simulink model "Top_Level_Model_arch"  (R2023a)
settings: Solver=VariableStepAuto  StartTime=0.0  StopTime=10.0  RelTol=1e-3
settings Model: Creator=hunte  LastModifiedBy=hunte

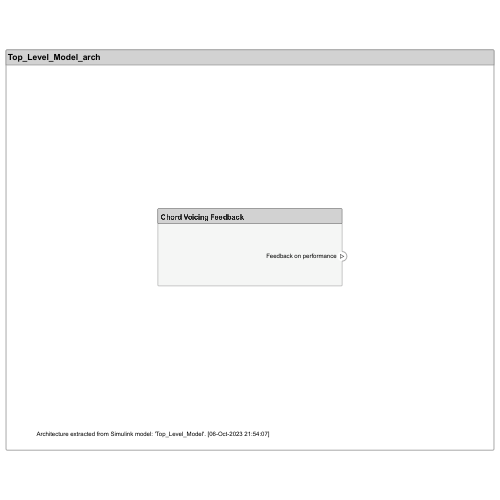
[thumbnail: Simulink's stored preview of the top-level diagram]
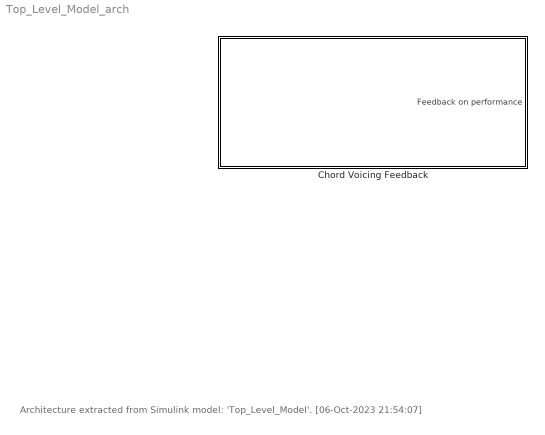
== system Top_Level_Model_arch ==
  note: Architecture extracted from Simulink model: 'Top_Level_Model'. [06-Oct-2023 21:54:07]
  "Chord Voicing Feedback " : Subsystem
      settings: PortSchema="{\"entries\":[{\"content\":{\"headerSize\":26,\"margin\":15,\"minimumSpacing\":25,\"sides\":[{\"content\":{},\"type\":\"ConnectorPlacement.EquallySpacedRectSide\",\"uuid\":\"aa7799b5-9463-4594-9ae2-36d4855ee31b\"},{\"content\":{\"connectorIds\":[\"Out1\"],\"side\":\"RIGHT\"},\"type\":\"ConnectorPlacement.EquallySpacedRectSide\",\"uuid\":\"2092a70f-f0fd-429a-8afe-090859a2b818\"},{\"content\":{\"side\":\"TOP\"},\"type\":\"ConnectorPlacement.EquallySpacedRectSide\",\"uuid\":\"da8f9889-6f26-4414-a897-b29829a1673f\"}]},\"type\":\"ConnectorPlacement.EquallySpacedConnector\",\"uuid\":\"7a26612b-cf01-40dc-98f5-e18304675eaa\"}],\"packageUris\":[\"http://schema.mathworks.com/mf0/Connector/R2020b\"],\"version\":\"1.0\"}"

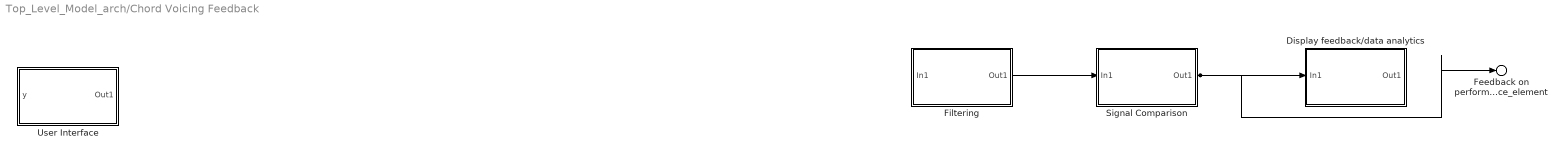
== system Top_Level_Model_arch/Chord Voicing Feedback  ==
  Display feedback/data analytics : Subsystem
      settings: PortSchema="{\"entries\":[{\"content\":{\"headerSize\":26,\"margin\":15,\"minimumSpacing\":25,\"sides\":[{\"content\":{\"connectorIds\":[\"In1\"]},\"type\":\"ConnectorPlacement.EquallySpacedRectSide\",\"uuid\":\"aa7799b5-9463-4594-9ae2-36d4855ee31b\"},{\"content\":{\"connectorIds\":[\"Out1\"],\"side\":\"RIGHT\"},\"type\":\"ConnectorPlacement.EquallySpacedRectSide\",\"uuid\":\"2092a70f-f0fd-429a-8afe-090859a2b818\"},{\"content\":{\"side\":\"TOP\"},\"type\":\"ConnectorPlacement.EquallySpacedRectSide\",\"uuid\":\"da8f9889-6f26-4414-a897-b29829a1673f\"}]},\"type\":\"ConnectorPlacement.EquallySpacedConnector\",\"uuid\":\"7a26612b-cf01-40dc-98f5-e18304675eaa\"}],\"packageUris\":[\"http://schema.mathworks.com/mf0/Connector/R2020b\"],\"version\":\"1.0\"}"
  Filtering : Subsystem
      settings: PortSchema="{\"entries\":[{\"content\":{\"headerSize\":26,\"margin\":15,\"minimumSpacing\":25,\"sides\":[{\"content\":{\"connectorIds\":[\"In1\"]},\"type\":\"ConnectorPlacement.EquallySpacedRectSide\",\"uuid\":\"aa7799b5-9463-4594-9ae2-36d4855ee31b\"},{\"content\":{\"connectorIds\":[\"Out1\"],\"side\":\"RIGHT\"},\"type\":\"ConnectorPlacement.EquallySpacedRectSide\",\"uuid\":\"2092a70f-f0fd-429a-8afe-090859a2b818\"},{\"content\":{\"side\":\"TOP\"},\"type\":\"ConnectorPlacement.EquallySpacedRectSide\",\"uuid\":\"da8f9889-6f26-4414-a897-b29829a1673f\"}]},\"type\":\"ConnectorPlacement.EquallySpacedConnector\",\"uuid\":\"7a26612b-cf01-40dc-98f5-e18304675eaa\"}],\"packageUris\":[\"http://schema.mathworks.com/mf0/Connector/R2020b\"],\"version\":\"1.0\"}"
  Signal Comparison : Subsystem
      settings: PortSchema="{\"entries\":[{\"content\":{\"headerSize\":26,\"margin\":15,\"minimumSpacing\":25,\"sides\":[{\"content\":{\"connectorIds\":[\"In1\"]},\"type\":\"ConnectorPlacement.EquallySpacedRectSide\",\"uuid\":\"aa7799b5-9463-4594-9ae2-36d4855ee31b\"},{\"content\":{\"connectorIds\":[\"Out1\"],\"side\":\"RIGHT\"},\"type\":\"ConnectorPlacement.EquallySpacedRectSide\",\"uuid\":\"2092a70f-f0fd-429a-8afe-090859a2b818\"},{\"content\":{\"side\":\"TOP\"},\"type\":\"ConnectorPlacement.EquallySpacedRectSide\",\"uuid\":\"da8f9889-6f26-4414-a897-b29829a1673f\"}]},\"type\":\"ConnectorPlacement.EquallySpacedConnector\",\"uuid\":\"7a26612b-cf01-40dc-98f5-e18304675eaa\"}],\"packageUris\":[\"http://schema.mathworks.com/mf0/Connector/R2020b\"],\"version\":\"1.0\"}"
  User Interface : Subsystem
      settings: PortSchema="{\"entries\":[{\"content\":{\"headerSize\":26,\"margin\":15,\"minimumSpacing\":25,\"sides\":[{\"content\":{\"connectorIds\":[\"In1\"]},\"type\":\"ConnectorPlacement.EquallySpacedRectSide\",\"uuid\":\"aa7799b5-9463-4594-9ae2-36d4855ee31b\"},{\"content\":{\"connectorIds\":[\"Out1\"],\"side\":\"RIGHT\"},\"type\":\"ConnectorPlacement.EquallySpacedRectSide\",\"uuid\":\"2092a70f-f0fd-429a-8afe-090859a2b818\"},{\"content\":{\"side\":\"TOP\"},\"type\":\"ConnectorPlacement.EquallySpacedRectSide\",\"uuid\":\"da8f9889-6f26-4414-a897-b29829a1673f\"}]},\"type\":\"ConnectorPlacement.EquallySpacedConnector\",\"uuid\":\"7a26612b-cf01-40dc-98f5-e18304675eaa\"}],\"packageUris\":[\"http://schema.mathworks.com/mf0/Connector/R2020b\"],\"version\":\"1.0\"}"
  Feedback on performance_element : Outport  PortName=Feedback on performance
  wires:
  Signal Comparison/1(Out1) -> Display feedback/data analytics/1(In1), Feedback on performance_element/1
  Filtering/1(Out1) -> Signal Comparison/1(In1)

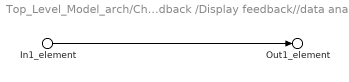
== system Top_Level_Model_arch/Chord Voicing Feedback /Display feedback//data analytics ==
  In1_element : Inport  PortName=In1
  Out1_element : Outport  PortName=Out1
  wires:
  In1_element/1 -> Out1_element/1

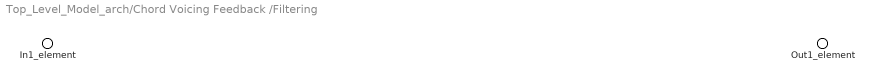
== system Top_Level_Model_arch/Chord Voicing Feedback /Filtering ==
  In1_element : Inport  PortName=In1
  Out1_element : Outport  PortName=Out1

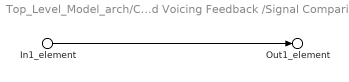
== system Top_Level_Model_arch/Chord Voicing Feedback /Signal Comparison ==
  In1_element : Inport  PortName=In1
  Out1_element : Outport  PortName=Out1
  wires:
  In1_element/1 -> Out1_element/1

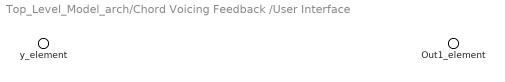
== system Top_Level_Model_arch/Chord Voicing Feedback /User Interface ==
  y_element : Inport  PortName=y
  Out1_element : Outport  PortName=Out1
